simulink model "VisionVehicleDetector"  (R2024b)
settings: Solver=FixedStepAuto  StartTime=0.0  StopTime=Inf  RelTol=1e-3  EnableMultiTasking=on
undefined symbols (not defined in the file): camera
libraries: visionanalysis x1
settings Model: Creator=The MathWorks, Inc.  LastModifiedBy=Lee
settings SolverCC: AlgebraicLoopSolver=TrustRegion  MaxZcPerStep=1
settings DataIOCC: SaveOutput=off  SaveTime=off  ReturnWorkspaceOutputs=off
settings OptimizationCC: DefaultParameterBehavior=Inlined  InlineInvariantSignals=on  EnhancedBackFolding=on  PassReuseOutputArgsAs=Individual arguments  ZeroExternalMemoryAtStartup=off  ZeroInternalMemoryAtStartup=off  InitFltsAndDblsToZero=on  EfficientFloat2IntCast=on  OptimizeBlockOrder=speed  DifferentSizesBufferReuse=on  OptimizationCustomize=off  EfficientTunableParamExpr=on
settings DebuggingCC: ParameterPrecisionLossMsg=none  ParameterTunabilityLossMsg=error  UnconnectedInputMsg=warning  UnconnectedOutputMsg=warning  UnconnectedLineMsg=warning  PregeneratedLibrarySubsystemCodeDiagnostic=none  SubsystemReferenceDiagnosticForUnitTest=warning  ArithmeticOperatorsInVariantConditions=warning
settings HardwareCC: ProdLongLongMode=on  TargetLongLongMode=on
settings ModelReferenceCC: EnableRefExpFcnMdlSchedulingChecks=on  PropagateVarSize=During execution
settings SFSimCC: SimUseLocalCustomCode=off
settings RTWCC: Description=Embedded Coder  SystemTargetFile=ert.tlc  TemplateMakefile=ert_default_tmf  RTWVerbose=off  RTWUseLocalCustomCode=off  BuildConfiguration=Faster Runs  CodeExecutionProfiling=on  CodeProfilingSaveOptions=AllData  TargetLang=C++  GPUComputeCapability=3.5  DLArmComputeVersion=19.05
settings CodeAppCC: ForceParamTrailComments=on  IgnoreCustomStorageClasses=off  OperatorAnnotations=on  SimulinkDataObjDesc=on  SFDataObjDesc=on  CustomSymbolStrGlobalVar=$N$M  CustomSymbolStrType=$N$M_T  CustomSymbolStrFcn=APV_$N$M$F  CustomSymbolStrMacro=$N$M  InsertBlockDesc=on
settings ERTTargetCC: TargetLangStandard=C++03 (ISO)  GenerateSampleERTMain=on  CombineSignalStateStructs=on  CodeInterfacePackaging=C++ class  SupportVariableSizeSignals=on  RootIOFormat=Structure reference  ERTCustomFileTemplate=example_file_process.tlc  DynamicArrayContainerType=coder::array
settings ConfigComp: CovScope=ReferencedModels  CovIncludeTopModel=off

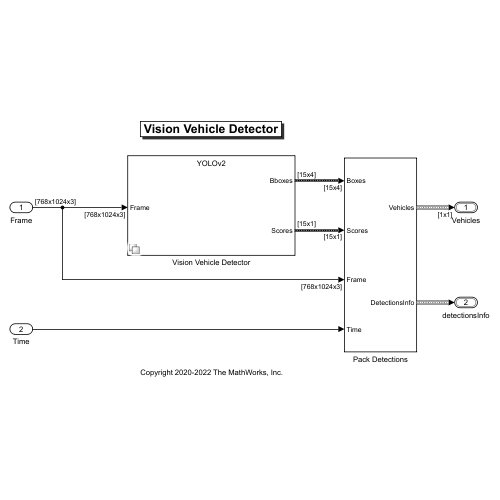
[thumbnail: Simulink's stored preview of the top-level diagram]
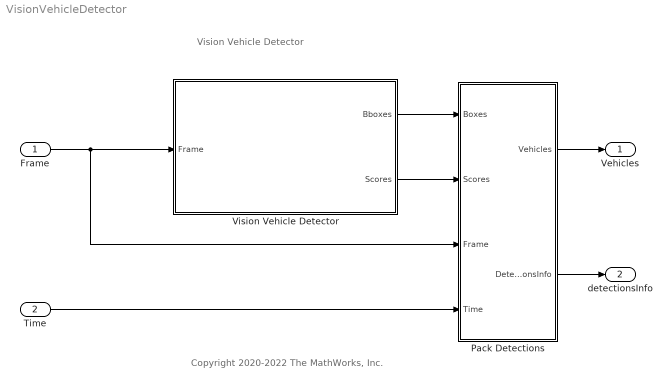
== system VisionVehicleDetector ==
  note: Copyright 2020-2022 The MathWorks, Inc.
  note: Vision Vehicle Detector
  Frame : Inport  OutDataTypeStr=uint8  PortDimensions=[camera.NumRows camera.NumColumns 3]  SampleTime=[0.10000000000000001,0]
  Time : Inport  Port=2  OutDataTypeStr=double  PortDimensions=1  SampleTime=[0.10000000000000001,0]
  Pack Detections : Subsystem
  Vision Vehicle Detector : Subsystem  Variant=on  VariantControl=Choice
  Vehicles : Outport  OutDataTypeStr=Bus: BusVision  PortDimensions=[1 1]  SampleTime=[0.10000000000000001,0]  BusOutputAsStruct=on
  detectionsInfo : Outport  Port=2  OutDataTypeStr=Bus: BusVisionInfo  BusOutputAsStruct=on
  wires:
  Time/1 -> Pack Detections/4(Time)
  Frame/1 -> Vision Vehicle Detector/1(Frame), Pack Detections/3(Frame)
  Pack Detections/1(Vehicles) -> Vehicles/1
  Vision Vehicle Detector/1(Bboxes) -> Pack Detections/1(Boxes)
  Pack Detections/2(DetectionsInfo) -> detectionsInfo/1
  Vision Vehicle Detector/2(Scores) -> Pack Detections/2(Scores)

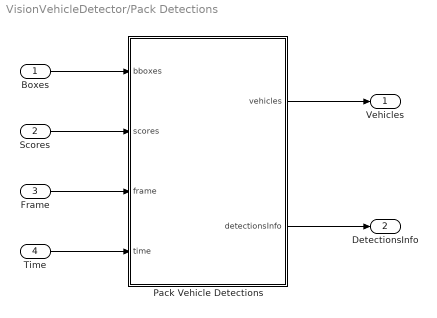
== system VisionVehicleDetector/Pack Detections ==
  Boxes : Inport
  Scores : Inport  Port=2
  Frame : Inport  Port=3
  Time : Inport  Port=4
  Pack Vehicle Detections : MATLAB Function  TreatAsAtomicUnit=on  mask{vehiclesOutputStruct=Simulink.Bus.createMATLABStruct('BusVision'), detectionsInfoOutputStruct=Simulink.Bus.createMATLABStruct('BusVisionInfo'), camera=camera, enableDisplay=off}
      mask prompts: vehiclesOutputStruct "Vehicles Output Struct"; detectionsInfoOutputStruct "Detections Info Output Struct"; enableDisplay "Enable Display"
  Vehicles : Outport
  DetectionsInfo : Outport  Port=2
  wires:
  Boxes/1 -> Pack Vehicle Detections/1(bboxes)
  Pack Vehicle Detections/1(vehicles) -> Vehicles/1
  Scores/1 -> Pack Vehicle Detections/2(scores)
  Pack Vehicle Detections/2(detectionsInfo) -> DetectionsInfo/1
  Frame/1 -> Pack Vehicle Detections/3(frame)
  Time/1 -> Pack Vehicle Detections/4(time)

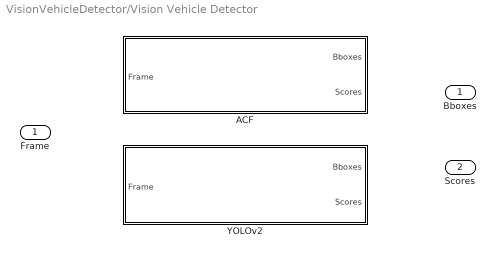
== system VisionVehicleDetector/Vision Vehicle Detector ==
  Frame : Inport
  ACF : Subsystem  VariantControl="detectorVariant == \"ACF\""
  YOLOv2 : Subsystem  VariantControl="detectorVariant == \"YOLOv2\""
  Bboxes : Outport
  Scores : Outport  Port=2

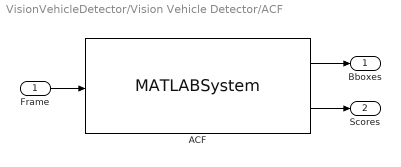
== system VisionVehicleDetector/Vision Vehicle Detector/ACF ==
  Frame : Inport
  ACF : MATLABSystem  System=HelperACFVehicleDetector  Camera=camera  MaxDetections=15  ACFModel=acfDetectorStruct  SimulateUsing=Interpreted execution
      mask Type: HelperACFVehicleDetector
      mask Display:
      | disp('HelperACFVehicleDetector');
      | port_label('input',1,'frame');
      | port_label('output',1,'bboxes');
      | port_label('output',2,'scores');
  Bboxes : Outport
  Scores : Outport  Port=2
  wires:
  Frame/1 -> ACF/1
  ACF/1 -> Bboxes/1
  ACF/2 -> Scores/1

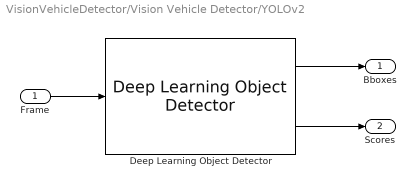
== system VisionVehicleDetector/Vision Vehicle Detector/YOLOv2 ==
  Frame : Inport
  Deep Learning Object Detector : visionanalysis/Deep Learning Object Detector  Detector=Detector from MATLAB function  DetectorFunction=vehicleDetectorYOLOv2  DetectorFilePath=C:\Users\rsuresh\OneDrive - MathWorks\Desktop\VVDDetect23a\vehicleDetectorYOLOv2Model.mat  MaxDetections=15  Bboxes=on  Scores=on  UseROI=on  AutoResize=on  ROI=[1 1 camera.ImageSize(2) round(camera.ImageSize(1)*0.678)]  Threshold=0.4  NumStrongestRegions=2000  UseMinSize=off  MinSize=[1 1]  UseMaxSize=off  MaxSize=[50 50]  ForceInterpretedSim=off
  Bboxes : Outport
  Scores : Outport  Port=2
  wires:
  Frame/1 -> Deep Learning Object Detector/1
  Deep Learning Object Detector/1 -> Bboxes/1
  Deep Learning Object Detector/2 -> Scores/1

== matlab function VisionVehicleDetector/Pack Detections/Pack Vehicle Detections ==
  data: bboxes input; vehicles output Bus: BusVision; scores input; frame input; time input; detectionsInfo output Bus: BusVisionInfo; vehiclesOutputStruct parameter; detectionsInfoOutputStruct parameter; camera parameter; enableDisplay parameter
function [vehicles,detectionsInfo] = helperPackVehicleDetections(bboxes,scores,frame,time, vehiclesOutputStruct, detectionsInfoOutputStruct, camera, enableDisplay)
    % Initialise Outputs
    vehicles = vehiclesOutputStruct;
    detectionsInfo = detectionsInfoOutputStruct;
    frameWithOverlays = frame;

    % Remove false positives
    [bboxes,scores] = selectStrongestBbox(bboxes,scores,"RatioType","Min","OverlapThreshold",0.4);

    % Define deployable video player for display vehicle detections
    persistent depVideoPlayer
    if isempty(depVideoPlayer) 
        depVideoPlayer = vision.DeployableVideoPlayer(Name='Vehicle Detections');
    end

    
    % Define Mono Camera sensor
    persistent sensor;
    if isempty(sensor)
        % Compute the camera intrinsics
        camIntrinsics = cameraIntrinsics(camera.FocalLength,camera.PrincipalPoint, camera.ImageSize);
        % Initialize the monocamera sensor
        sensor = monoCamera(camIntrinsics, camera.Position(3),'Pitch', camera.Rotation(2));
    end

    % Compute the vehicle location in vehicle coordinates and pack outputs
    if ~isempty(bboxes)
        sensorOut         = detectVehicles(bboxes,scores,sensor);
        vehicles          = packVehicleDetections(vehiclesOutputStruct,sensorOut,camera,time);
        detectionsInfo    = packDetectionsInfo(detectionsInfoOutputStruct,sensorOut);
        frameWithOverlays = overlaySensorOutputs(frame, sensorOut);
    end
    
    % Display vehicle detections
    if enableDisplay == true
        depVideoPlayer(frameWithOverlays);
    end
end
%-------------------------------------------------------------------------%
% Supporting Functions
%-------------------------------------------------------------------------%
function sensorOut =  detectVehicles(bboxes,scores,sensor)
    % Compute distance in vehicle coordinates
    locations = zeros(size(bboxes,1),2);
    for i = 1:size(bboxes, 1)
        bbox  = bboxes(i, :);
        
        yBottom = bbox(2) + bbox(4) - 1;
        xCenter = bbox(1) + (bbox(3)-1)/2;
        
        locations(i,:) = imageToVehicle(sensor, [xCenter, yBottom]);
    end
    sensorOut.vehicleLocations = locations;
    sensorOut.vehicleBoxes     = bboxes;
    sensorOut.vehicleScores    = scores;
end
%-------------------------------------------------------------------------%
function vehicles = packVehicleDetections(outputStruct,sensorOut,camera,t)
    %Initialize detections bus with zeros.
    vehicles = outputStruct;     
    
    locations = sensorOut.vehicleLocations;
    
    numDetections = size(locations,1);
    vehicles.NumDetections = numDetections;
    
    for n = 1:numDetections
        % Bias location measurements as expected by sensor fusion -
        % Sensor fusion is with respect to vehicle center with
        % Unreal sensors.
        %  - camera.PositionSim3D is mount position
        % with respect to vehicle center.
        locations(n,:) = locations(n,:) + camera.PositionSim3d(1:2);
        
        % Pack to constant velocity measurement format:
        vehicles.IsValidTime = true;
        vehicles.Detections(n).Measurement = [...
                                                locations(n,1),...
                                                locations(n,2),...
                                                0]'; % [x,y,z]
        vehicles.Detections(n).MeasurementNoise = camera.MeasurementNoise;
        vehicles.Detections(n).Time(:)       = t;
        vehicles.Detections(n).SensorIndex   = 1;
        vehicles.Detections(n).ObjectClassID = 1;
        vehicles.Detections(n).MeasurementParameters.Frame = drivingCoordinateFrameType.Rectangular;
        vehicles.Detections(n).MeasurementParameters.HasVelocity = false;
        vehicles.Detections(n).MeasurementParameters.Orientation = eye(3);
    end
end
%-------------------------------------------------------------------------%
function detectionsInfo = packDetectionsInfo(outputStruct,sensorOut)
    detectionsInfo = outputStruct;
    detectionsInfo.NumDetections = size(sensorOut.vehicleLocations,1);
    for n = 1:detectionsInfo.NumDetections
        detectionsInfo.Detections(n).Boxes  = [sensorOut.vehicleBoxes(n,1) sensorOut.vehicleBoxes(n,2) sensorOut.vehicleBoxes(n,3) sensorOut.vehicleBoxes(n,4)];
        detectionsInfo.Detections(n).Scores  = double(sensorOut.vehicleScores(n));
    end
end
%-------------------------------------------------------------------------%
function frameWithOverlays = overlaySensorOutputs(frame, sensorOut)
    locations  = sensorOut.vehicleLocations;
    bboxes     = sensorOut.vehicleBoxes;
    imgOut     = frame;
    for i = 1:size(locations, 1)
        location = locations(i, :);
        bbox     = bboxes(i, :);
        label    = sprintf('X=%0.2f, Y=%0.2f', location(1), location(2));
        imgOut   = insertObjectAnnotation(imgOut,'rectangle', bbox, label);
    end
    frameWithOverlays = imgOut;
end
